simulink model "Q11"  (R2021b)
settings: Solver=VariableStepAuto  StartTime=0.0  StopTime=10.0  RelTol=1e-3
undefined symbols (not defined in the file): deadbeat, G, H, observer
settings Model: Creator=Siavash  LastModifiedBy=Siavash

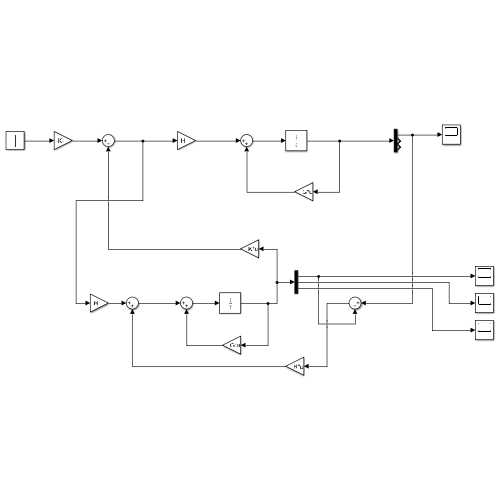
[thumbnail: Simulink's stored preview of the top-level diagram]
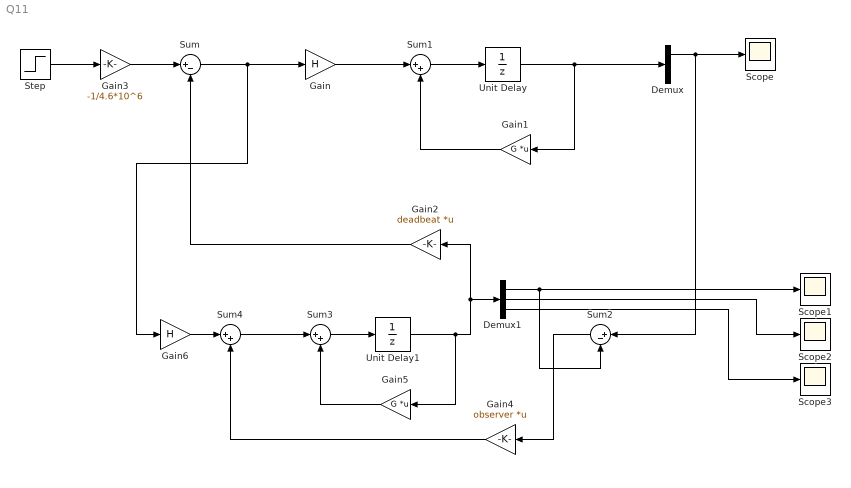
== system Q11 ==
  Demux : Demux  Outputs=3
  Demux1 : Demux  Outputs=3
  Gain : Gain  Gain=H
  Gain1 : Gain  Gain=G  Multiplication=Matrix(K*u)
  Gain2 : Gain  Gain=deadbeat  Multiplication=Matrix(K*u)
  Gain3 : Gain  Gain=-1/4.6*10^6
  Gain4 : Gain  Gain=observer  Multiplication=Matrix(K*u)
  Gain5 : Gain  Gain=G  Multiplication=Matrix(K*u)
  Gain6 : Gain  Gain=H
  Scope{,1..3} (4 alike) : Scope
  Step : Step  SampleTime=0
  Sum : Sum  Inputs=|+-
  Sum1 : Sum  Inputs=|++
  Sum2 : Sum  Inputs=|+-
  Sum3 : Sum  Inputs=|++
  Sum4 : Sum  Inputs=|++
  Unit Delay : UnitDelay  SampleTime=-1  HasFrameUpgradeWarning=on
  Unit Delay1 : UnitDelay  SampleTime=-1  HasFrameUpgradeWarning=on
  wires:
  Sum/1 -> Gain6/1, Gain/1
  Gain/1 -> Sum1/1
  Sum1/1 -> Unit Delay/1
  Gain1/1 -> Sum1/2
  Unit Delay/1 -> Demux/1, Gain1/1
  Gain2/1 -> Sum/2
  Demux/1 -> Scope/1, Sum2/1
  Step/1 -> Gain3/1
  Gain3/1 -> Sum/1
  Sum2/1 -> Gain4/1
  Unit Delay1/1 -> Gain5/1, Gain2/1, Demux1/1
  Sum3/1 -> Unit Delay1/1
  Gain5/1 -> Sum3/2
  Sum4/1 -> Sum3/1
  Gain4/1 -> Sum4/2
  Demux1/1 -> Sum2/2, Scope1/1
  Gain6/1 -> Sum4/1
  Demux1/2 -> Scope2/1
  Demux1/3 -> Scope3/1
